simulink model "test_linearpll_selfwork"  (R2018b)
settings: Solver=ode4  StartTime=0.0  StopTime=0.12  FixedStep=0.01/44100  RelTol=1e-3
values from neighbouring files (symbols this model uses):
  a = k0/2    (= 50000)    [projectcode final version.m]
  amp = k0/kvco    [projectcode final version.m]
  kf = df/(max (x))    [projectcode final version.m]
  kvco = 2*pi*kf    [projectcode final version.m]
settings Model: Creator=HsuWeiChe  LastModifiedBy=yangq

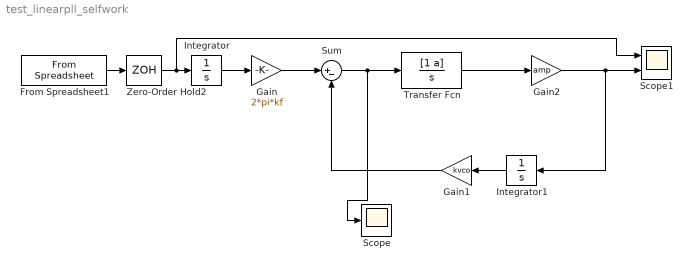
== system test_linearpll_selfwork ==
  From Spreadsheet1 : FromSpreadsheet  FileName=audio.xlsx  TreatFirstColumnAs=Data  SampleTime=1/44100
  Gain : Gain  Gain=2*pi*kf
  Gain1 : Gain  Gain=kvco
  Gain2 : Gain  Gain=amp
  Integrator : Integrator
  Integrator1 : Integrator
  Scope : Scope
  Scope1 : Scope  NumInputPorts=2
  Sum : Sum  Inputs=|+-
  Transfer Fcn : TransferFcn  Numerator=[1 a]  Denominator=[1 0]
  Zero-Order Hold2 : ZeroOrderHold  SampleTime=1/44100
  wires:
  Zero-Order Hold2/1 -> Scope1/1, Integrator/1
  From Spreadsheet1/1 -> Zero-Order Hold2/1
  Integrator/1 -> Gain/1
  Sum/1 -> Scope/1, Transfer Fcn/1
  Transfer Fcn/1 -> Gain2/1
  Integrator1/1 -> Gain1/1
  Gain2/1 -> Integrator1/1, Scope1/2
  Gain1/1 -> Sum/2
  Gain/1 -> Sum/1
